simulink model "Online_Ordering_System_Functional_Architecture"  (R2025a)
settings: Solver=VariableStepAuto  StartTime=0.0  StopTime=10.0  RelTol=1e-3
model workspace (MAT data in the model file):
  Data = Simulink.Bus
  Data.Alignment = -1
  Data.PreserveElementDimensions = 0
  Data.Elements_internal(1) = Simulink.BusElement
  Data.Elements_internal(1).Min_internal = 30000
  Data.Elements_internal(1).Max_internal = 50000
  Data.Elements_internal(1).DimensionsMode = 'Fixed'
  Data.Elements_internal(1).SamplingMode = 'Sample based'
  Data.Elements_internal(1).SampleTime = -1
  Data.Elements_internal(1).Description = 'Person'
  Data.Elements_internal(1).DocUnits = '30000'
  Data.Elements_internal(1).Name = 'TargetUser'
  Data.Elements_internal(1).DataType_internal = 'single'
  Data.Elements_internal(1).Complexity = 'real'
  Data.Elements_internal(1).Dimensions = 1
  Data.Elements_internal(2) = Simulink.BusElement
  Data.Elements_internal(2).Min_internal = 10000
  Data.Elements_internal(2).Max_internal = 50000
  Data.Elements_internal(2).DimensionsMode = 'Fixed'
  Data.Elements_internal(2).SamplingMode = 'Sample based'
  Data.Elements_internal(2).SampleTime = -1
  Data.Elements_internal(2).Description = 'Person'
  Data.Elements_internal(2).DocUnits = '10000'
  Data.Elements_internal(2).Name = 'TargetPartner'
  Data.Elements_internal(2).DataType_internal = 'single'
  Data.Elements_internal(2).Complexity = 'real'
  Data.Elements_internal(2).Dimensions = 1
  Data.Elements_internal(3) = Simulink.BusElement
  Data.Elements_internal(3).Min_internal = 1
  Data.Elements_internal(3).Max_internal = 2
  Data.Elements_internal(3).DimensionsMode = 'Fixed'
  Data.Elements_internal(3).SamplingMode = 'Sample based'
  Data.Elements_internal(3).SampleTime = -1
  Data.Elements_internal(3).Description = 'Second'
  Data.Elements_internal(3).DocUnits = '2s'
  Data.Elements_internal(3).Name = 'ResponseTime'
  Data.Elements_internal(3).DataType_internal = 'single'
  Data.Elements_internal(3).Complexity = 'real'
  Data.Elements_internal(3).Dimensions = 1
  Data.Elements_internal(4) = Simulink.BusElement
  Data.Elements_internal(4).Min_internal = 1
  Data.Elements_internal(4).Max_internal = 5
  Data.Elements_internal(4).DimensionsMode = 'Fixed'
  Data.Elements_internal(4).SamplingMode = 'Sample based'
  Data.Elements_internal(4).SampleTime = -1
  Data.Elements_internal(4).Description = 'Second'
  Data.Elements_internal(4).DocUnits = '5s'
  Data.Elements_internal(4).Name = 'ProcessTime'
  Data.Elements_internal(4).DataType_internal = 'single'
  Data.Elements_internal(4).Complexity = 'real'
  Data.Elements_internal(4).Dimensions = 1
  Data.DataScope = 'Auto'
  ValueType = Simulink.ValueType
(part 1 of 2)
settings Model: Creator=OdaNobuyuki  LastModifiedBy=annic

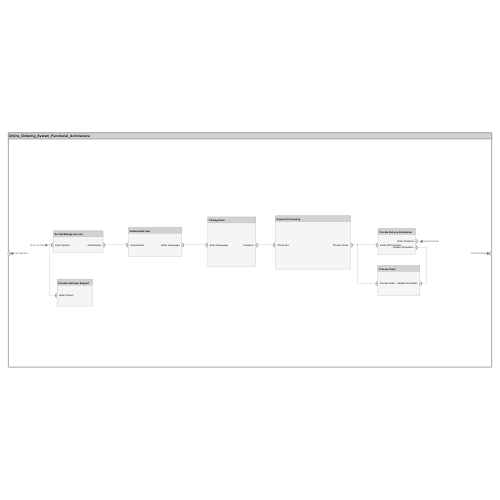
[thumbnail: Simulink's stored preview of the top-level diagram]
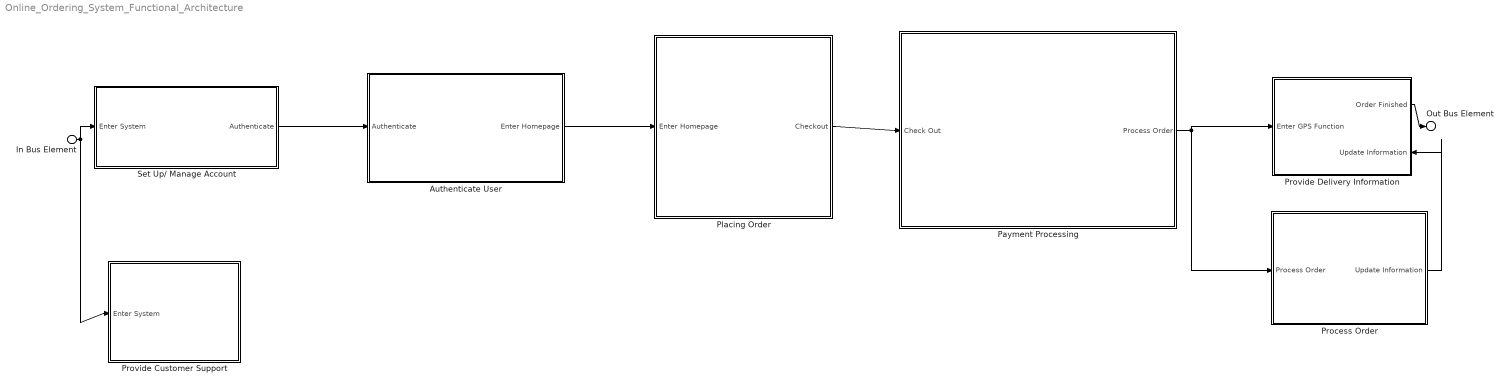
== system Online_Ordering_System_Functional_Architecture ==
  In Bus Element : Inport  PortName=Enter System
  "Authenticate User " : Subsystem
      settings: PortSchema="{\"entries\":[{\"content\":{\"headerSize\":26,\"margin\":15,\"minimumSpacing\":25,\"sides\":[{\"content\":{\"connectorIds\":[\"In1\"]},\"type\":\"ConnectorPlacement.EquallySpacedRectSide\",\"uuid\":\"427d1f3e-23ef-431e-830a-8ee80d1c0343\"},{\"content\":{\"connectorIds\":[\"Out1\"],\"side\":\"RIGHT\"},\"type\":\"ConnectorPlacement.EquallySpacedRectSide\",\"uuid\":\"a94733dc-dc80-40b7-a069-e69a5f529ec8\"},{\"content\":{\"side\":\"TOP\"},\"type\":\"ConnectorPlacement.EquallySpacedRectSide\",\"uuid\":\"aab6e856-7d0a-4bba-a547-38d5d593c589\"}]},\"type\":\"ConnectorPlacement.EquallySpacedConnector\",\"uuid\":\"17eb8191-1c5c-46d9-ae9e-c0a8464555a8\"}],\"packageUris\":[\"http://schema.mathworks.com/mf0/Connector/R2020b\"],\"version\":\"1.0\"}"
  Payment Processing : Subsystem
      settings: PortSchema="{\"entries\":[{\"content\":{\"headerSize\":26,\"margin\":15,\"minimumSpacing\":25,\"sides\":[{\"content\":{\"connectorIds\":[\"In1\"]},\"type\":\"ConnectorPlacement.EquallySpacedRectSide\",\"uuid\":\"427d1f3e-23ef-431e-830a-8ee80d1c0343\"},{\"content\":{\"connectorIds\":[\"Out1\"],\"side\":\"RIGHT\"},\"type\":\"ConnectorPlacement.EquallySpacedRectSide\",\"uuid\":\"a94733dc-dc80-40b7-a069-e69a5f529ec8\"},{\"content\":{\"side\":\"TOP\"},\"type\":\"ConnectorPlacement.EquallySpacedRectSide\",\"uuid\":\"aab6e856-7d0a-4bba-a547-38d5d593c589\"},{\"content\":{\"side\":\"BOTTOM\"},\"type\":\"ConnectorPlacement.EquallySpacedRectSide\",\"uuid\":\"c3292acf-2eb6-42cd-a4a7-82302ef25f03\"}]},\"type\":\"ConnectorPlacement.EquallySpacedConnector\",\"uuid\":\"17eb8191-1c5c-46d9-ae9e-c0a8464555a8\"}],\"packageUris\":[\"http://schema.mathworks.com/mf0/Connector/R2020b\"],\"version\":\"1.0\"}"
  Placing Order : Subsystem
      settings: PortSchema="{\"entries\":[{\"content\":{\"headerSize\":26,\"margin\":15,\"minimumSpacing\":25,\"sides\":[{\"content\":{\"connectorIds\":[\"In1\"]},\"type\":\"ConnectorPlacement.EquallySpacedRectSide\",\"uuid\":\"427d1f3e-23ef-431e-830a-8ee80d1c0343\"},{\"content\":{\"connectorIds\":[\"Out1\"],\"side\":\"RIGHT\"},\"type\":\"ConnectorPlacement.EquallySpacedRectSide\",\"uuid\":\"a94733dc-dc80-40b7-a069-e69a5f529ec8\"},{\"content\":{\"side\":\"TOP\"},\"type\":\"ConnectorPlacement.EquallySpacedRectSide\",\"uuid\":\"aab6e856-7d0a-4bba-a547-38d5d593c589\"},{\"content\":{\"side\":\"BOTTOM\"},\"type\":\"ConnectorPlacement.EquallySpacedRectSide\",\"uuid\":\"a89a1022-ae61-47b7-80bc-ebacb029706c\"}]},\"type\":\"ConnectorPlacement.EquallySpacedConnector\",\"uuid\":\"17eb8191-1c5c-46d9-ae9e-c0a8464555a8\"}],\"packageUris\":[\"http://schema.mathworks.com/mf0/Connector/R2020b\"],\"version\":\"1.0\"}"
  "Process Order " : Subsystem
      settings: PortSchema="{\"entries\":[{\"content\":{\"headerSize\":26,\"margin\":15,\"minimumSpacing\":25,\"sides\":[{\"content\":{\"connectorIds\":[\"In1\"]},\"type\":\"ConnectorPlacement.EquallySpacedRectSide\",\"uuid\":\"d2ebed04-42f4-4bd6-aa56-c214d37abe86\"},{\"content\":{\"connectorIds\":[\"Out1\"],\"side\":\"RIGHT\"},\"type\":\"ConnectorPlacement.EquallySpacedRectSide\",\"uuid\":\"0a328130-2da5-4535-b8fd-dee261bd04a3\"},{\"content\":{\"side\":\"TOP\"},\"type\":\"ConnectorPlacement.EquallySpacedRectSide\",\"uuid\":\"410ea5eb-e20b-4523-bb7e-a86253749ceb\"}]},\"type\":\"ConnectorPlacement.EquallySpacedConnector\",\"uuid\":\"5600d62f-d466-4629-981b-50f24b9b11a3\"}],\"packageUris\":[\"http://schema.mathworks.com/mf0/Connector/R2020b\"],\"version\":\"1.0\"}"
  Provide Customer Support : Subsystem
      settings: PortSchema="{\"entries\":[{\"content\":{\"headerSize\":26,\"margin\":15,\"minimumSpacing\":25,\"sides\":[{\"content\":{\"connectorIds\":[\"In1\"]},\"type\":\"ConnectorPlacement.EquallySpacedRectSide\",\"uuid\":\"427d1f3e-23ef-431e-830a-8ee80d1c0343\"},{\"content\":{\"side\":\"RIGHT\"},\"type\":\"ConnectorPlacement.EquallySpacedRectSide\",\"uuid\":\"a94733dc-dc80-40b7-a069-e69a5f529ec8\"},{\"content\":{\"side\":\"TOP\"},\"type\":\"ConnectorPlacement.EquallySpacedRectSide\",\"uuid\":\"aab6e856-7d0a-4bba-a547-38d5d593c589\"},{\"content\":{\"side\":\"BOTTOM\"},\"type\":\"ConnectorPlacement.EquallySpacedRectSide\",\"uuid\":\"351d9b7c-52a6-4554-b5b1-677764f6b427\"}]},\"type\":\"ConnectorPlacement.EquallySpacedConnector\",\"uuid\":\"17eb8191-1c5c-46d9-ae9e-c0a8464555a8\"}],\"packageUris\":[\"http://schema.mathworks.com/mf0/Connector/R2020b\"],\"version\":\"1.0\"}"
  Provide Delivery Information : Subsystem
      settings: PortSchema="{\"entries\":[{\"content\":{\"headerSize\":26,\"margin\":15,\"minimumSpacing\":25,\"sides\":[{\"content\":{\"connectorIds\":[\"In2\"]},\"type\":\"ConnectorPlacement.EquallySpacedRectSide\",\"uuid\":\"d2ebed04-42f4-4bd6-aa56-c214d37abe86\"},{\"content\":{\"connectorIds\":[\"Out1\",\"In1\"],\"side\":\"RIGHT\"},\"type\":\"ConnectorPlacement.EquallySpacedRectSide\",\"uuid\":\"0a328130-2da5-4535-b8fd-dee261bd04a3\"},{\"content\":{\"side\":\"TOP\"},\"type\":\"ConnectorPlacement.EquallySpacedRectSide\",\"uuid\":\"410ea5eb-e20b-4523-bb7e-a86253749ceb\"},{\"content\":{\"side\":\"BOTTOM\"},\"type\":\"ConnectorPlacement.EquallySpacedRectSide\",\"uuid\":\"443981ea-c855-4245-98e1-85cb0d225c25\"}]},\"type\":\"ConnectorPlacement.EquallySpacedConnector\",\"uuid\":\"5600d62f-d466-4629-981b-50f24b9b11a3\"}],\"packageUris\":[\"http://schema.mathworks.com/mf0/Connector/R2020b\"],\"version\":\"1.0\"}"
  Set Up/ Manage Account : Subsystem
      settings: PortSchema="{\"entries\":[{\"content\":{\"headerSize\":26,\"margin\":15,\"minimumSpacing\":25,\"sides\":[{\"content\":{\"connectorIds\":[\"In1\"]},\"type\":\"ConnectorPlacement.EquallySpacedRectSide\",\"uuid\":\"47f10906-199a-4fc3-b50f-b8829921055b\"},{\"content\":{\"connectorIds\":[\"Out1\"],\"side\":\"RIGHT\"},\"type\":\"ConnectorPlacement.EquallySpacedRectSide\",\"uuid\":\"92935151-f687-4cd9-918a-4edbdcb1ae87\"},{\"content\":{\"side\":\"TOP\"},\"type\":\"ConnectorPlacement.EquallySpacedRectSide\",\"uuid\":\"015ac99b-8cf7-4451-a810-2c7151c004f5\"}]},\"type\":\"ConnectorPlacement.EquallySpacedConnector\",\"uuid\":\"2d28be76-8335-46d7-935d-5d2731314622\"}],\"packageUris\":[\"http://schema.mathworks.com/mf0/Connector/R2020b\"],\"version\":\"1.0\"}"
  Out Bus Element : Outport  PortName=Order Finished
  wires:
  "Authenticate User "/1(Enter Homepage) -> Placing Order/1(Enter Homepage)
  Placing Order/1(Checkout) -> Payment Processing/1(Check Out)
  Payment Processing/1(Process Order) -> "Process Order "/1(Process Order), Provide Delivery Information/2(Enter GPS Function)
  In Bus Element/1 -> Provide Customer Support/1(Enter System), Set Up/ Manage Account/1(Enter System)
  Set Up/ Manage Account/1(Authenticate) -> "Authenticate User "/1(Authenticate)
  Provide Delivery Information/1(Order Finished) -> Out Bus Element/1
  "Process Order "/1(Update Information) -> Provide Delivery Information/1(Update Information)

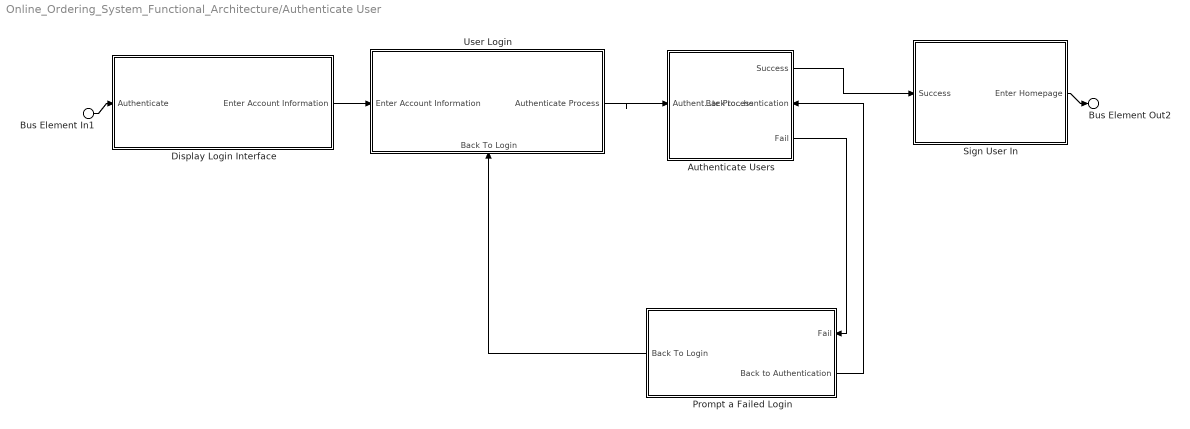
== system Online_Ordering_System_Functional_Architecture/Authenticate User  ==
  Bus Element In1 : Inport  PortName=Authenticate
  Authenticate Users : Subsystem
      settings: PortSchema="{\"entries\":[{\"content\":{\"headerSize\":26,\"margin\":15,\"minimumSpacing\":25,\"sides\":[{\"content\":{\"connectorIds\":[\"In2\"]},\"type\":\"ConnectorPlacement.EquallySpacedRectSide\",\"uuid\":\"427d1f3e-23ef-431e-830a-8ee80d1c0343\"},{\"content\":{\"connectorIds\":[\"Out1\",\"In1\",\"Out2\"],\"side\":\"RIGHT\"},\"type\":\"ConnectorPlacement.EquallySpacedRectSide\",\"uuid\":\"a94733dc-dc80-40b7-a069-e69a5f529ec8\"},{\"content\":{\"side\":\"TOP\"},\"type\":\"ConnectorPlacement.EquallySpacedRectSide\",\"uuid\":\"aab6e856-7d0a-4bba-a547-38d5d593c589\"},{\"content\":{\"side\":\"BOTTOM\"},\"type\":\"ConnectorPlacement.EquallySpacedRectSide\",\"uuid\":\"822edfb6-5de7-4787-92bc-976e01cc291a\"}]},\"type\":\"ConnectorPlacement.EquallySpacedConnector\",\"uuid\":\"17eb8191-1c5c-46d9-ae9e-c0a8464555a8\"}],\"packageUris\":[\"http://schema.mathworks.com/mf0/Connector/R2020b\"],\"version\":\"1.0\"}"
  Display Login Interface : Subsystem
      settings: PortSchema="{\"entries\":[{\"content\":{\"headerSize\":26,\"margin\":15,\"minimumSpacing\":25,\"sides\":[{\"content\":{\"connectorIds\":[\"In1\"]},\"type\":\"ConnectorPlacement.EquallySpacedRectSide\",\"uuid\":\"cbb74984-7595-4789-b046-96ead26edeb9\"},{\"content\":{\"connectorIds\":[\"Out1\"],\"side\":\"RIGHT\"},\"type\":\"ConnectorPlacement.EquallySpacedRectSide\",\"uuid\":\"b6bb8368-8099-4b12-9d55-2c29ae804ffc\"},{\"content\":{\"side\":\"TOP\"},\"type\":\"ConnectorPlacement.EquallySpacedRectSide\",\"uuid\":\"14a6774e-c600-4f70-83e3-a7d0c3cf7479\"},{\"content\":{\"side\":\"BOTTOM\"},\"type\":\"ConnectorPlacement.EquallySpacedRectSide\",\"uuid\":\"deb2294e-400e-4f84-ba24-f2715792f4b9\"}]},\"type\":\"ConnectorPlacement.EquallySpacedConnector\",\"uuid\":\"469ef3cc-c012-4ecc-a677-bf3638dfce1b\"}],\"packageUris\":[\"http://schema.mathworks.com/mf0/Connector/R2020b\"],\"version\":\"1.0\"}"
  Prompt a Failed Login : Subsystem
      settings: PortSchema="{\"entries\":[{\"content\":{\"headerSize\":26,\"margin\":15,\"minimumSpacing\":25,\"sides\":[{\"content\":{\"connectorIds\":[\"Out1\"]},\"type\":\"ConnectorPlacement.EquallySpacedRectSide\",\"uuid\":\"427d1f3e-23ef-431e-830a-8ee80d1c0343\"},{\"content\":{\"connectorIds\":[\"In1\",\"Out2\"],\"side\":\"RIGHT\"},\"type\":\"ConnectorPlacement.EquallySpacedRectSide\",\"uuid\":\"a94733dc-dc80-40b7-a069-e69a5f529ec8\"},{\"content\":{\"side\":\"TOP\"},\"type\":\"ConnectorPlacement.EquallySpacedRectSide\",\"uuid\":\"aab6e856-7d0a-4bba-a547-38d5d593c589\"}]},\"type\":\"ConnectorPlacement.EquallySpacedConnector\",\"uuid\":\"17eb8191-1c5c-46d9-ae9e-c0a8464555a8\"}],\"packageUris\":[\"http://schema.mathworks.com/mf0/Connector/R2020b\"],\"version\":\"1.0\"}"
  Sign User In : Subsystem
      settings: PortSchema="{\"entries\":[{\"content\":{\"headerSize\":26,\"margin\":15,\"minimumSpacing\":25,\"sides\":[{\"content\":{\"connectorIds\":[\"In1\"]},\"type\":\"ConnectorPlacement.EquallySpacedRectSide\",\"uuid\":\"427d1f3e-23ef-431e-830a-8ee80d1c0343\"},{\"content\":{\"connectorIds\":[\"Out1\"],\"side\":\"RIGHT\"},\"type\":\"ConnectorPlacement.EquallySpacedRectSide\",\"uuid\":\"a94733dc-dc80-40b7-a069-e69a5f529ec8\"},{\"content\":{\"side\":\"TOP\"},\"type\":\"ConnectorPlacement.EquallySpacedRectSide\",\"uuid\":\"aab6e856-7d0a-4bba-a547-38d5d593c589\"},{\"content\":{\"side\":\"BOTTOM\"},\"type\":\"ConnectorPlacement.EquallySpacedRectSide\",\"uuid\":\"4782b0d4-0180-487e-b6f5-72f073cbe76a\"}]},\"type\":\"ConnectorPlacement.EquallySpacedConnector\",\"uuid\":\"17eb8191-1c5c-46d9-ae9e-c0a8464555a8\"}],\"packageUris\":[\"http://schema.mathworks.com/mf0/Connector/R2020b\"],\"version\":\"1.0\"}"
  "User Login " : Subsystem
      settings: PortSchema="{\"entries\":[{\"content\":{\"headerSize\":26,\"margin\":15,\"minimumSpacing\":25,\"sides\":[{\"content\":{\"connectorIds\":[\"In2\"]},\"type\":\"ConnectorPlacement.EquallySpacedRectSide\",\"uuid\":\"d2ebed04-42f4-4bd6-aa56-c214d37abe86\"},{\"content\":{\"connectorIds\":[\"Out1\"],\"side\":\"RIGHT\"},\"type\":\"ConnectorPlacement.EquallySpacedRectSide\",\"uuid\":\"0a328130-2da5-4535-b8fd-dee261bd04a3\"},{\"content\":{\"side\":\"TOP\"},\"type\":\"ConnectorPlacement.EquallySpacedRectSide\",\"uuid\":\"410ea5eb-e20b-4523-bb7e-a86253749ceb\"},{\"content\":{\"connectorIds\":[\"In1\"],\"side\":\"BOTTOM\"},\"type\":\"ConnectorPlacement.EquallySpacedRectSide\",\"uuid\":\"388ab0ab-6a87-40e3-b544-46c520a133d8\"}]},\"type\":\"ConnectorPlacement.EquallySpacedConnector\",\"uuid\":\"5600d62f-d466-4629-981b-50f24b9b11a3\"}],\"packageUris\":[\"http://schema.mathworks.com/mf0/Connector/R2020b\"],\"version\":\"1.0\"}"
  Bus Element Out2 : Outport  PortName=Enter Homepage
  wires:
  Authenticate Users/1(Success) -> Sign User In/1(Success)
  Display Login Interface/1(Enter Account Information) -> "User Login "/2(Enter Account Information)
  Prompt a Failed Login/2(Back to Authentication) -> Authenticate Users/1(Back to Authentication)
  "User Login "/1(Authenticate Process) -> Authenticate Users/2(Authenticate Process)
  Prompt a Failed Login/1(Back To Login) -> "User Login "/1(Back To Login)
  Sign User In/1(Enter Homepage) -> Bus Element Out2/1
  Bus Element In1/1 -> Display Login Interface/1(Authenticate)
  Authenticate Users/2(Fail) -> Prompt a Failed Login/1(Fail)

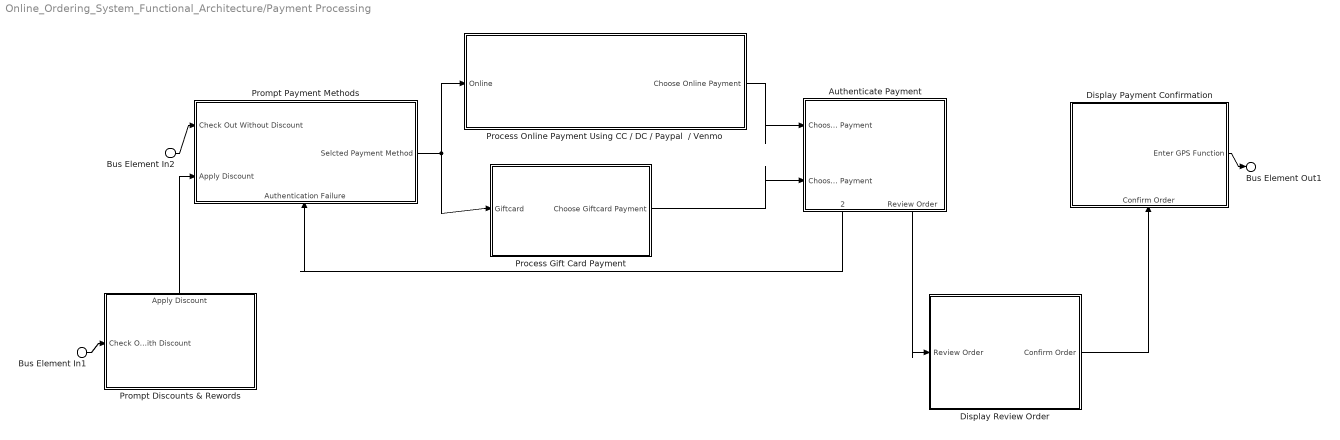
== system Online_Ordering_System_Functional_Architecture/Payment Processing ==
  Bus Element In1 : Inport  PortName=Check Out
  Bus Element In2 : Inport  PortName=Check Out
  Authenticate Payment : Subsystem
      settings: PortSchema="{\"entries\":[{\"content\":{\"headerSize\":26,\"margin\":15,\"minimumSpacing\":25,\"sides\":[{\"content\":{\"connectorIds\":[\"In1\",\"In2\"]},\"type\":\"ConnectorPlacement.EquallySpacedRectSide\",\"uuid\":\"427d1f3e-23ef-431e-830a-8ee80d1c0343\"},{\"content\":{\"side\":\"RIGHT\"},\"type\":\"ConnectorPlacement.EquallySpacedRectSide\",\"uuid\":\"a94733dc-dc80-40b7-a069-e69a5f529ec8\"},{\"content\":{\"side\":\"TOP\"},\"type\":\"ConnectorPlacement.EquallySpacedRectSide\",\"uuid\":\"aab6e856-7d0a-4bba-a547-38d5d593c589\"},{\"content\":{\"connectorIds\":[\"Out2\",\"Out1\"],\"side\":\"BOTTOM\"},\"type\":\"ConnectorPlacement.EquallySpacedRectSide\",\"uuid\":\"2134340b-1a1d-4804-aa4c-47d156557184\"}]},\"type\":\"ConnectorPlacement.EquallySpacedConnector\",\"uuid\":\"17eb8191-1c5c-46d9-ae9e-c0a8464555a8\"}],\"packageUris\":[\"http://schema.mathworks.com/mf0/Connector/R2020b\"],\"version\":\"1.0\"}"
  Display Payment Confirmation : Subsystem
      settings: PortSchema="{\"entries\":[{\"content\":{\"headerSize\":26,\"margin\":15,\"minimumSpacing\":25,\"sides\":[{\"content\":{},\"type\":\"ConnectorPlacement.EquallySpacedRectSide\",\"uuid\":\"cbb74984-7595-4789-b046-96ead26edeb9\"},{\"content\":{\"connectorIds\":[\"Out1\"],\"side\":\"RIGHT\"},\"type\":\"ConnectorPlacement.EquallySpacedRectSide\",\"uuid\":\"b6bb8368-8099-4b12-9d55-2c29ae804ffc\"},{\"content\":{\"side\":\"TOP\"},\"type\":\"ConnectorPlacement.EquallySpacedRectSide\",\"uuid\":\"14a6774e-c600-4f70-83e3-a7d0c3cf7479\"},{\"content\":{\"connectorIds\":[\"In1\"],\"side\":\"BOTTOM\"},\"type\":\"ConnectorPlacement.EquallySpacedRectSide\",\"uuid\":\"a82d93e2-79e4-4503-92a2-65c1f83a9361\"}]},\"type\":\"ConnectorPlacement.EquallySpacedConnector\",\"uuid\":\"469ef3cc-c012-4ecc-a677-bf3638dfce1b\"}],\"packageUris\":[\"http://schema.mathworks.com/mf0/Connector/R2020b\"],\"version\":\"1.0\"}"
  Display Review Order : Subsystem
      settings: PortSchema="{\"entries\":[{\"content\":{\"headerSize\":26,\"margin\":15,\"minimumSpacing\":25,\"sides\":[{\"content\":{\"connectorIds\":[\"In1\"]},\"type\":\"ConnectorPlacement.EquallySpacedRectSide\",\"uuid\":\"47f10906-199a-4fc3-b50f-b8829921055b\"},{\"content\":{\"connectorIds\":[\"Out1\"],\"side\":\"RIGHT\"},\"type\":\"ConnectorPlacement.EquallySpacedRectSide\",\"uuid\":\"92935151-f687-4cd9-918a-4edbdcb1ae87\"},{\"content\":{\"side\":\"TOP\"},\"type\":\"ConnectorPlacement.EquallySpacedRectSide\",\"uuid\":\"015ac99b-8cf7-4451-a810-2c7151c004f5\"}]},\"type\":\"ConnectorPlacement.EquallySpacedConnector\",\"uuid\":\"2d28be76-8335-46d7-935d-5d2731314622\"}],\"packageUris\":[\"http://schema.mathworks.com/mf0/Connector/R2020b\"],\"version\":\"1.0\"}"
  Process Gift Card Payment : Subsystem
      settings: PortSchema="{\"entries\":[{\"content\":{\"headerSize\":26,\"margin\":15,\"minimumSpacing\":25,\"sides\":[{\"content\":{\"connectorIds\":[\"In1\"]},\"type\":\"ConnectorPlacement.EquallySpacedRectSide\",\"uuid\":\"427d1f3e-23ef-431e-830a-8ee80d1c0343\"},{\"content\":{\"connectorIds\":[\"Out1\"],\"side\":\"RIGHT\"},\"type\":\"ConnectorPlacement.EquallySpacedRectSide\",\"uuid\":\"a94733dc-dc80-40b7-a069-e69a5f529ec8\"},{\"content\":{\"side\":\"TOP\"},\"type\":\"ConnectorPlacement.EquallySpacedRectSide\",\"uuid\":\"aab6e856-7d0a-4bba-a547-38d5d593c589\"}]},\"type\":\"ConnectorPlacement.EquallySpacedConnector\",\"uuid\":\"17eb8191-1c5c-46d9-ae9e-c0a8464555a8\"}],\"packageUris\":[\"http://schema.mathworks.com/mf0/Connector/R2020b\"],\"version\":\"1.0\"}"
  Process Online Payment Using CC / DC / Paypal  / Venmo : Subsystem
      settings: PortSchema="{\"entries\":[{\"content\":{\"headerSize\":26,\"margin\":15,\"minimumSpacing\":25,\"sides\":[{\"content\":{\"connectorIds\":[\"In1\"]},\"type\":\"ConnectorPlacement.EquallySpacedRectSide\",\"uuid\":\"427d1f3e-23ef-431e-830a-8ee80d1c0343\"},{\"content\":{\"connectorIds\":[\"Out1\"],\"side\":\"RIGHT\"},\"type\":\"ConnectorPlacement.EquallySpacedRectSide\",\"uuid\":\"a94733dc-dc80-40b7-a069-e69a5f529ec8\"},{\"content\":{\"side\":\"TOP\"},\"type\":\"ConnectorPlacement.EquallySpacedRectSide\",\"uuid\":\"aab6e856-7d0a-4bba-a547-38d5d593c589\"}]},\"type\":\"ConnectorPlacement.EquallySpacedConnector\",\"uuid\":\"17eb8191-1c5c-46d9-ae9e-c0a8464555a8\"}],\"packageUris\":[\"http://schema.mathworks.com/mf0/Connector/R2020b\"],\"version\":\"1.0\"}"
  Prompt Discounts & Rewords : Subsystem
      settings: PortSchema="{\"entries\":[{\"content\":{\"headerSize\":26,\"margin\":15,\"minimumSpacing\":25,\"sides\":[{\"content\":{\"connectorIds\":[\"In1\"]},\"type\":\"ConnectorPlacement.EquallySpacedRectSide\",\"uuid\":\"427d1f3e-23ef-431e-830a-8ee80d1c0343\"},{\"content\":{\"side\":\"RIGHT\"},\"type\":\"ConnectorPlacement.EquallySpacedRectSide\",\"uuid\":\"a94733dc-dc80-40b7-a069-e69a5f529ec8\"},{\"content\":{\"connectorIds\":[\"Out1\"],\"side\":\"TOP\"},\"type\":\"ConnectorPlacement.EquallySpacedRectSide\",\"uuid\":\"aab6e856-7d0a-4bba-a547-38d5d593c589\"}]},\"type\":\"ConnectorPlacement.EquallySpacedConnector\",\"uuid\":\"17eb8191-1c5c-46d9-ae9e-c0a8464555a8\"}],\"packageUris\":[\"http://schema.mathworks.com/mf0/Connector/R2020b\"],\"version\":\"1.0\"}"
  Prompt Payment Methods : Subsystem
      settings: PortSchema="{\"entries\":[{\"content\":{\"headerSize\":26,\"margin\":15,\"minimumSpacing\":25,\"sides\":[{\"content\":{\"connectorIds\":[\"In1\",\"In2\"]},\"type\":\"ConnectorPlacement.EquallySpacedRectSide\",\"uuid\":\"427d1f3e-23ef-431e-830a-8ee80d1c0343\"},{\"content\":{\"connectorIds\":[\"Out1\"],\"side\":\"RIGHT\"},\"type\":\"ConnectorPlacement.EquallySpacedRectSide\",\"uuid\":\"a94733dc-dc80-40b7-a069-e69a5f529ec8\"},{\"content\":{\"side\":\"TOP\"},\"type\":\"ConnectorPlacement.EquallySpacedRectSide\",\"uuid\":\"aab6e856-7d0a-4bba-a547-38d5d593c589\"},{\"content\":{\"connectorIds\":[\"In3\"],\"side\":\"BOTTOM\"},\"type\":\"ConnectorPlacement.EquallySpacedRectSide\",\"uuid\":\"301fbdec-26db-4103-a088-b13178cf7d4f\"}]},\"type\":\"ConnectorPlacement.EquallySpacedConnector\",\"uuid\":\"17eb8191-1c5c-46d9-ae9e-c0a8464555a8\"}],\"packageUris\":[\"http://schema.mathworks.com/mf0/Connector/R2020b\"],\"version\":\"1.0\"}"
  Bus Element Out1 : Outport  PortName=Process Order
  wires:
  Prompt Payment Methods/1(Selcted Payment Method) -> Process Online Payment Using CC / DC / Paypal  / Venmo/1(Online), Process Gift Card Payment/1(Giftcard)
  Process Online Payment Using CC / DC / Paypal  / Venmo/1(Choose Online Payment) -> Authenticate Payment/1(Choose Online Payment)
  Process Gift Card Payment/1(Choose Giftcard Payment) -> Authenticate Payment/2(Choose Giftcard Payment)
  Authenticate Payment/2(Authentication Failure) -> Prompt Payment Methods/3(Authentication Failure)
  Bus Element In1/1 -> Prompt Discounts & Rewords/1(Check Out With Discount)
  Prompt Discounts & Rewords/1(Apply Discount) -> Prompt Payment Methods/2(Apply Discount)
  Bus Element In2/1 -> Prompt Payment Methods/1(Check Out Without Discount)
  Authenticate Payment/1(Review Order) -> Display Review Order/1(Review Order)
  Display Review Order/1(Confirm Order) -> Display Payment Confirmation/1(Confirm Order)
  Display Payment Confirmation/1(Enter GPS Function) -> Bus Element Out1/1

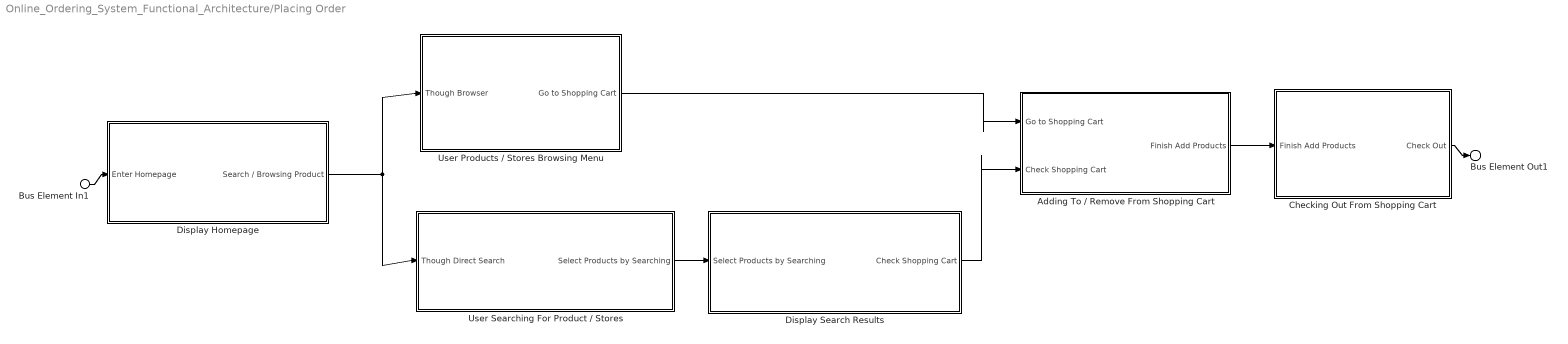
== system Online_Ordering_System_Functional_Architecture/Placing Order ==
  Bus Element In1 : Inport  PortName=Enter Homepage
  "Adding To / Remove From Shopping Cart " : Subsystem
      settings: PortSchema="{\"entries\":[{\"content\":{\"headerSize\":26,\"margin\":15,\"minimumSpacing\":25,\"sides\":[{\"content\":{\"connectorIds\":[\"In1\",\"In2\"]},\"type\":\"ConnectorPlacement.EquallySpacedRectSide\",\"uuid\":\"427d1f3e-23ef-431e-830a-8ee80d1c0343\"},{\"content\":{\"connectorIds\":[\"Out1\"],\"side\":\"RIGHT\"},\"type\":\"ConnectorPlacement.EquallySpacedRectSide\",\"uuid\":\"a94733dc-dc80-40b7-a069-e69a5f529ec8\"},{\"content\":{\"side\":\"TOP\"},\"type\":\"ConnectorPlacement.EquallySpacedRectSide\",\"uuid\":\"aab6e856-7d0a-4bba-a547-38d5d593c589\"},{\"content\":{\"side\":\"BOTTOM\"},\"type\":\"ConnectorPlacement.EquallySpacedRectSide\",\"uuid\":\"b903f41b-b4dc-49c0-8a4d-a823a8bb045a\"}]},\"type\":\"ConnectorPlacement.EquallySpacedConnector\",\"uuid\":\"17eb8191-1c5c-46d9-ae9e-c0a8464555a8\"}],\"packageUris\":[\"http://schema.mathworks.com/mf0/Connector/R2020b\"],\"version\":\"1.0\"}"
  Checking Out From Shopping Cart : Subsystem
      settings: PortSchema="{\"entries\":[{\"content\":{\"headerSize\":26,\"margin\":15,\"minimumSpacing\":25,\"sides\":[{\"content\":{\"connectorIds\":[\"In1\"]},\"type\":\"ConnectorPlacement.EquallySpacedRectSide\",\"uuid\":\"d2ebed04-42f4-4bd6-aa56-c214d37abe86\"},{\"content\":{\"connectorIds\":[\"Out1\"],\"side\":\"RIGHT\"},\"type\":\"ConnectorPlacement.EquallySpacedRectSide\",\"uuid\":\"0a328130-2da5-4535-b8fd-dee261bd04a3\"},{\"content\":{\"side\":\"TOP\"},\"type\":\"ConnectorPlacement.EquallySpacedRectSide\",\"uuid\":\"410ea5eb-e20b-4523-bb7e-a86253749ceb\"}]},\"type\":\"ConnectorPlacement.EquallySpacedConnector\",\"uuid\":\"5600d62f-d466-4629-981b-50f24b9b11a3\"}],\"packageUris\":[\"http://schema.mathworks.com/mf0/Connector/R2020b\"],\"version\":\"1.0\"}"
  Display Homepage : Subsystem
      settings: PortSchema="{\"entries\":[{\"content\":{\"headerSize\":26,\"margin\":15,\"minimumSpacing\":25,\"sides\":[{\"content\":{\"connectorIds\":[\"In1\"]},\"type\":\"ConnectorPlacement.EquallySpacedRectSide\",\"uuid\":\"cbb74984-7595-4789-b046-96ead26edeb9\"},{\"content\":{\"connectorIds\":[\"Out1\"],\"side\":\"RIGHT\"},\"type\":\"ConnectorPlacement.EquallySpacedRectSide\",\"uuid\":\"b6bb8368-8099-4b12-9d55-2c29ae804ffc\"},{\"content\":{\"side\":\"TOP\"},\"type\":\"ConnectorPlacement.EquallySpacedRectSide\",\"uuid\":\"14a6774e-c600-4f70-83e3-a7d0c3cf7479\"},{\"content\":{\"side\":\"BOTTOM\"},\"type\":\"ConnectorPlacement.EquallySpacedRectSide\",\"uuid\":\"d057ab6e-a0b6-4baa-a98f-672ff88698d4\"}]},\"type\":\"ConnectorPlacement.EquallySpacedConnector\",\"uuid\":\"469ef3cc-c012-4ecc-a677-bf3638dfce1b\"}],\"packageUris\":[\"http://schema.mathworks.com/mf0/Connector/R2020b\"],\"version\":\"1.0\"}"
  Display Search Results : Subsystem
      settings: PortSchema="{\"entries\":[{\"content\":{\"headerSize\":26,\"margin\":15,\"minimumSpacing\":25,\"sides\":[{\"content\":{\"connectorIds\":[\"In1\"]},\"type\":\"ConnectorPlacement.EquallySpacedRectSide\",\"uuid\":\"cbb74984-7595-4789-b046-96ead26edeb9\"},{\"content\":{\"connectorIds\":[\"Out1\"],\"side\":\"RIGHT\"},\"type\":\"ConnectorPlacement.EquallySpacedRectSide\",\"uuid\":\"b6bb8368-8099-4b12-9d55-2c29ae804ffc\"},{\"content\":{\"side\":\"TOP\"},\"type\":\"ConnectorPlacement.EquallySpacedRectSide\",\"uuid\":\"14a6774e-c600-4f70-83e3-a7d0c3cf7479\"},{\"content\":{\"side\":\"BOTTOM\"},\"type\":\"ConnectorPlacement.EquallySpacedRectSide\",\"uuid\":\"96a52d4b-311b-45a3-8c8a-5b70822256d6\"}]},\"type\":\"ConnectorPlacement.EquallySpacedConnector\",\"uuid\":\"469ef3cc-c012-4ecc-a677-bf3638dfce1b\"}],\"packageUris\":[\"http://schema.mathworks.com/mf0/Connector/R2020b\"],\"version\":\"1.0\"}"
  User Products / Stores Browsing Menu : Subsystem
      settings: PortSchema="{\"entries\":[{\"content\":{\"headerSize\":26,\"margin\":15,\"minimumSpacing\":25,\"sides\":[{\"content\":{\"connectorIds\":[\"In1\"]},\"type\":\"ConnectorPlacement.EquallySpacedRectSide\",\"uuid\":\"427d1f3e-23ef-431e-830a-8ee80d1c0343\"},{\"content\":{\"connectorIds\":[\"Out1\"],\"side\":\"RIGHT\"},\"type\":\"ConnectorPlacement.EquallySpacedRectSide\",\"uuid\":\"a94733dc-dc80-40b7-a069-e69a5f529ec8\"},{\"content\":{\"side\":\"TOP\"},\"type\":\"ConnectorPlacement.EquallySpacedRectSide\",\"uuid\":\"aab6e856-7d0a-4bba-a547-38d5d593c589\"},{\"content\":{\"side\":\"BOTTOM\"},\"type\":\"ConnectorPlacement.EquallySpacedRectSide\",\"uuid\":\"06e25ceb-3515-4a34-9a5e-b52bdfde88f0\"}]},\"type\":\"ConnectorPlacement.EquallySpacedConnector\",\"uuid\":\"17eb8191-1c5c-46d9-ae9e-c0a8464555a8\"}],\"packageUris\":[\"http://schema.mathworks.com/mf0/Connector/R2020b\"],\"version\":\"1.0\"}"
  User Searching For Product / Stores : Subsystem
      settings: PortSchema="{\"entries\":[{\"content\":{\"headerSize\":26,\"margin\":15,\"minimumSpacing\":25,\"sides\":[{\"content\":{\"connectorIds\":[\"In1\"]},\"type\":\"ConnectorPlacement.EquallySpacedRectSide\",\"uuid\":\"427d1f3e-23ef-431e-830a-8ee80d1c0343\"},{\"content\":{\"connectorIds\":[\"Out1\"],\"side\":\"RIGHT\"},\"type\":\"ConnectorPlacement.EquallySpacedRectSide\",\"uuid\":\"a94733dc-dc80-40b7-a069-e69a5f529ec8\"},{\"content\":{\"side\":\"TOP\"},\"type\":\"ConnectorPlacement.EquallySpacedRectSide\",\"uuid\":\"aab6e856-7d0a-4bba-a547-38d5d593c589\"},{\"content\":{\"side\":\"BOTTOM\"},\"type\":\"ConnectorPlacement.EquallySpacedRectSide\",\"uuid\":\"442269c5-54c2-4a2e-b298-a7048d1c7a55\"}]},\"type\":\"ConnectorPlacement.EquallySpacedConnector\",\"uuid\":\"17eb8191-1c5c-46d9-ae9e-c0a8464555a8\"}],\"packageUris\":[\"http://schema.mathworks.com/mf0/Connector/R2020b\"],\"version\":\"1.0\"}"
  Bus Element Out1 : Outport  PortName=Checkout
  wires:
  Display Homepage/1(Search / Browsing Product) -> User Products / Stores Browsing Menu/1(Though Browser), User Searching For Product / Stores/1(Though Direct Search)
  User Searching For Product / Stores/1(Select Products by Searching) -> Display Search Results/1(Select Products by Searching)
  Display Search Results/1(Check Shopping Cart) -> "Adding To / Remove From Shopping Cart "/2(Check Shopping Cart)
  Bus Element In1/1 -> Display Homepage/1(Enter Homepage)
  User Products / Stores Browsing Menu/1(Go to Shopping Cart) -> "Adding To / Remove From Shopping Cart "/1(Go to Shopping Cart)
  "Adding To / Remove From Shopping Cart "/1(Finish Add Products) -> Checking Out From Shopping Cart/1(Finish Add Products)
  Checking Out From Shopping Cart/1(Check Out) -> Bus Element Out1/1

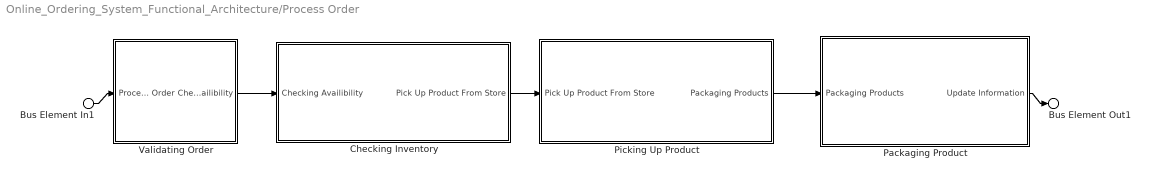
== system Online_Ordering_System_Functional_Architecture/Process Order  ==
  Bus Element In1 : Inport  PortName=Process Order
  Checking Inventory : Subsystem
      settings: PortSchema="{\"entries\":[{\"content\":{\"headerSize\":26,\"margin\":15,\"minimumSpacing\":25,\"sides\":[{\"content\":{\"connectorIds\":[\"In1\"]},\"type\":\"ConnectorPlacement.EquallySpacedRectSide\",\"uuid\":\"d2ebed04-42f4-4bd6-aa56-c214d37abe86\"},{\"content\":{\"connectorIds\":[\"Out1\"],\"side\":\"RIGHT\"},\"type\":\"ConnectorPlacement.EquallySpacedRectSide\",\"uuid\":\"0a328130-2da5-4535-b8fd-dee261bd04a3\"},{\"content\":{\"side\":\"TOP\"},\"type\":\"ConnectorPlacement.EquallySpacedRectSide\",\"uuid\":\"410ea5eb-e20b-4523-bb7e-a86253749ceb\"}]},\"type\":\"ConnectorPlacement.EquallySpacedConnector\",\"uuid\":\"5600d62f-d466-4629-981b-50f24b9b11a3\"}],\"packageUris\":[\"http://schema.mathworks.com/mf0/Connector/R2020b\"],\"version\":\"1.0\"}"
  Packaging Product : Subsystem
      settings: PortSchema="{\"entries\":[{\"content\":{\"headerSize\":26,\"margin\":15,\"minimumSpacing\":25,\"sides\":[{\"content\":{\"connectorIds\":[\"In1\"]},\"type\":\"ConnectorPlacement.EquallySpacedRectSide\",\"uuid\":\"d2ebed04-42f4-4bd6-aa56-c214d37abe86\"},{\"content\":{\"connectorIds\":[\"Out1\"],\"side\":\"RIGHT\"},\"type\":\"ConnectorPlacement.EquallySpacedRectSide\",\"uuid\":\"0a328130-2da5-4535-b8fd-dee261bd04a3\"},{\"content\":{\"side\":\"TOP\"},\"type\":\"ConnectorPlacement.EquallySpacedRectSide\",\"uuid\":\"410ea5eb-e20b-4523-bb7e-a86253749ceb\"}]},\"type\":\"ConnectorPlacement.EquallySpacedConnector\",\"uuid\":\"5600d62f-d466-4629-981b-50f24b9b11a3\"}],\"packageUris\":[\"http://schema.mathworks.com/mf0/Connector/R2020b\"],\"version\":\"1.0\"}"
  Picking Up Product : Subsystem
      settings: PortSchema="{\"entries\":[{\"content\":{\"headerSize\":26,\"margin\":15,\"minimumSpacing\":25,\"sides\":[{\"content\":{\"connectorIds\":[\"In1\"]},\"type\":\"ConnectorPlacement.EquallySpacedRectSide\",\"uuid\":\"d2ebed04-42f4-4bd6-aa56-c214d37abe86\"},{\"content\":{\"connectorIds\":[\"Out1\"],\"side\":\"RIGHT\"},\"type\":\"ConnectorPlacement.EquallySpacedRectSide\",\"uuid\":\"0a328130-2da5-4535-b8fd-dee261bd04a3\"},{\"content\":{\"side\":\"TOP\"},\"type\":\"ConnectorPlacement.EquallySpacedRectSide\",\"uuid\":\"410ea5eb-e20b-4523-bb7e-a86253749ceb\"}]},\"type\":\"ConnectorPlacement.EquallySpacedConnector\",\"uuid\":\"5600d62f-d466-4629-981b-50f24b9b11a3\"}],\"packageUris\":[\"http://schema.mathworks.com/mf0/Connector/R2020b\"],\"version\":\"1.0\"}"
  Validating Order : Subsystem
      settings: PortSchema="{\"entries\":[{\"content\":{\"headerSize\":26,\"margin\":15,\"minimumSpacing\":25,\"sides\":[{\"content\":{\"connectorIds\":[\"In1\"]},\"type\":\"ConnectorPlacement.EquallySpacedRectSide\",\"uuid\":\"d2ebed04-42f4-4bd6-aa56-c214d37abe86\"},{\"content\":{\"connectorIds\":[\"Out1\"],\"side\":\"RIGHT\"},\"type\":\"ConnectorPlacement.EquallySpacedRectSide\",\"uuid\":\"0a328130-2da5-4535-b8fd-dee261bd04a3\"},{\"content\":{\"side\":\"TOP\"},\"type\":\"ConnectorPlacement.EquallySpacedRectSide\",\"uuid\":\"410ea5eb-e20b-4523-bb7e-a86253749ceb\"}]},\"type\":\"ConnectorPlacement.EquallySpacedConnector\",\"uuid\":\"5600d62f-d466-4629-981b-50f24b9b11a3\"}],\"packageUris\":[\"http://schema.mathworks.com/mf0/Connector/R2020b\"],\"version\":\"1.0\"}"
  Bus Element Out1 : Outport  PortName=Update Information
  wires:
  Validating Order/1("Checking Availibility ") -> Checking Inventory/1("Checking Availibility ")
  Checking Inventory/1(Pick Up Product From Store) -> Picking Up Product/1(Pick Up Product From Store)
  Picking Up Product/1(Packaging Products) -> Packaging Product/1(Packaging Products)
  Packaging Product/1(Update Information) -> Bus Element Out1/1
  Bus Element In1/1 -> Validating Order/1(Process Order)

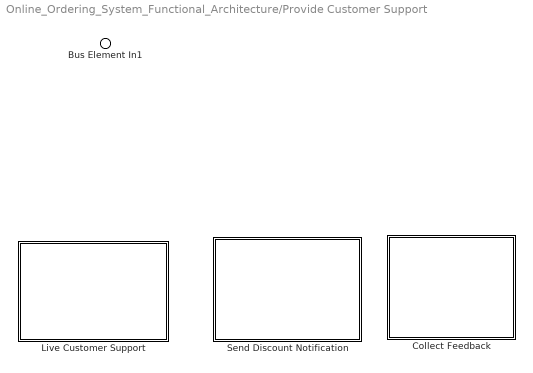
== system Online_Ordering_System_Functional_Architecture/Provide Customer Support ==
  Bus Element In1 : Inport  PortName=Enter System
  Collect Feedback : Subsystem
      settings: PortSchema="{\"entries\":[{\"content\":{\"headerSize\":26,\"margin\":15,\"minimumSpacing\":25,\"sides\":[{\"content\":{},\"type\":\"ConnectorPlacement.EquallySpacedRectSide\",\"uuid\":\"47f10906-199a-4fc3-b50f-b8829921055b\"},{\"content\":{\"side\":\"RIGHT\"},\"type\":\"ConnectorPlacement.EquallySpacedRectSide\",\"uuid\":\"92935151-f687-4cd9-918a-4edbdcb1ae87\"},{\"content\":{\"side\":\"TOP\"},\"type\":\"ConnectorPlacement.EquallySpacedRectSide\",\"uuid\":\"015ac99b-8cf7-4451-a810-2c7151c004f5\"},{\"content\":{\"side\":\"BOTTOM\"},\"type\":\"ConnectorPlacement.EquallySpacedRectSide\",\"uuid\":\"eec9be38-4ba6-426b-a1f1-2c37e91dc163\"}]},\"type\":\"ConnectorPlacement.EquallySpacedConnector\",\"uuid\":\"2d28be76-8335-46d7-935d-5d2731314622\"}],\"packageUris\":[\"http://schema.mathworks.com/mf0/Connector/R2020b\"],\"version\":\"1.0\"}"
  Live Customer Support : Subsystem
      settings: PortSchema="{\"entries\":[{\"content\":{\"headerSize\":26,\"margin\":15,\"minimumSpacing\":25,\"sides\":[{\"content\":{},\"type\":\"ConnectorPlacement.EquallySpacedRectSide\",\"uuid\":\"47f10906-199a-4fc3-b50f-b8829921055b\"},{\"content\":{\"side\":\"RIGHT\"},\"type\":\"ConnectorPlacement.EquallySpacedRectSide\",\"uuid\":\"92935151-f687-4cd9-918a-4edbdcb1ae87\"},{\"content\":{\"side\":\"TOP\"},\"type\":\"ConnectorPlacement.EquallySpacedRectSide\",\"uuid\":\"015ac99b-8cf7-4451-a810-2c7151c004f5\"},{\"content\":{\"side\":\"BOTTOM\"},\"type\":\"ConnectorPlacement.EquallySpacedRectSide\",\"uuid\":\"c8e12821-783c-47e1-bb50-05fb22703402\"}]},\"type\":\"ConnectorPlacement.EquallySpacedConnector\",\"uuid\":\"2d28be76-8335-46d7-935d-5d2731314622\"}],\"packageUris\":[\"http://schema.mathworks.com/mf0/Connector/R2020b\"],\"version\":\"1.0\"}"
  Send Discount Notification : Subsystem
      settings: PortSchema="{\"entries\":[{\"content\":{\"headerSize\":26,\"margin\":15,\"minimumSpacing\":25,\"sides\":[{\"content\":{},\"type\":\"ConnectorPlacement.EquallySpacedRectSide\",\"uuid\":\"47f10906-199a-4fc3-b50f-b8829921055b\"},{\"content\":{\"side\":\"RIGHT\"},\"type\":\"ConnectorPlacement.EquallySpacedRectSide\",\"uuid\":\"92935151-f687-4cd9-918a-4edbdcb1ae87\"},{\"content\":{\"side\":\"TOP\"},\"type\":\"ConnectorPlacement.EquallySpacedRectSide\",\"uuid\":\"015ac99b-8cf7-4451-a810-2c7151c004f5\"},{\"content\":{\"side\":\"BOTTOM\"},\"type\":\"ConnectorPlacement.EquallySpacedRectSide\",\"uuid\":\"ba1e2227-187e-420e-b74b-a66b6d876499\"}]},\"type\":\"ConnectorPlacement.EquallySpacedConnector\",\"uuid\":\"2d28be76-8335-46d7-935d-5d2731314622\"}],\"packageUris\":[\"http://schema.mathworks.com/mf0/Connector/R2020b\"],\"version\":\"1.0\"}"

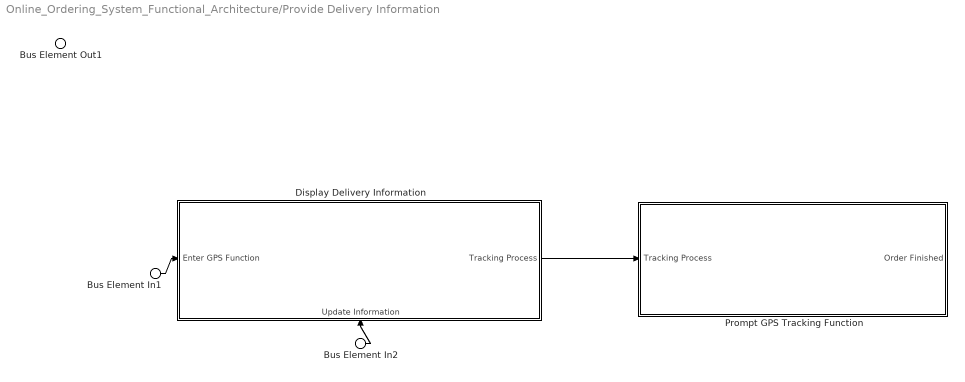
== system Online_Ordering_System_Functional_Architecture/Provide Delivery Information ==
  Bus Element In2 : Inport  PortName=Update Information
  Bus Element In1 : Inport  Port=2  PortName=Enter GPS Function
  Display Delivery Information : Subsystem
      settings: PortSchema="{\"entries\":[{\"content\":{\"headerSize\":26,\"margin\":15,\"minimumSpacing\":25,\"sides\":[{\"content\":{\"connectorIds\":[\"In2\"]},\"type\":\"ConnectorPlacement.EquallySpacedRectSide\",\"uuid\":\"427d1f3e-23ef-431e-830a-8ee80d1c0343\"},{\"content\":{\"connectorIds\":[\"Out1\"],\"side\":\"RIGHT\"},\"type\":\"ConnectorPlacement.EquallySpacedRectSide\",\"uuid\":\"a94733dc-dc80-40b7-a069-e69a5f529ec8\"},{\"content\":{\"side\":\"TOP\"},\"type\":\"ConnectorPlacement.EquallySpacedRectSide\",\"uuid\":\"aab6e856-7d0a-4bba-a547-38d5d593c589\"},{\"content\":{\"connectorIds\":[\"In1\"],\"side\":\"BOTTOM\"},\"type\":\"ConnectorPlacement.EquallySpacedRectSide\",\"uuid\":\"9b163a09-8a4d-4810-a0ad-ac99f601e974\"}]},\"type\":\"ConnectorPlacement.EquallySpacedConnector\",\"uuid\":\"17eb8191-1c5c-46d9-ae9e-c0a8464555a8\"}],\"packageUris\":[\"http://schema.mathworks.com/mf0/Connector/R2020b\"],\"version\":\"1.0\"}"
  Prompt GPS Tracking Function : Subsystem
      settings: PortSchema="{\"entries\":[{\"content\":{\"headerSize\":26,\"margin\":15,\"minimumSpacing\":25,\"sides\":[{\"content\":{\"connectorIds\":[\"In1\"]},\"type\":\"ConnectorPlacement.EquallySpacedRectSide\",\"uuid\":\"427d1f3e-23ef-431e-830a-8ee80d1c0343\"},{\"content\":{\"connectorIds\":[\"Out1\"],\"side\":\"RIGHT\"},\"type\":\"ConnectorPlacement.EquallySpacedRectSide\",\"uuid\":\"a94733dc-dc80-40b7-a069-e69a5f529ec8\"},{\"content\":{\"side\":\"TOP\"},\"type\":\"ConnectorPlacement.EquallySpacedRectSide\",\"uuid\":\"aab6e856-7d0a-4bba-a547-38d5d593c589\"}]},\"type\":\"ConnectorPlacement.EquallySpacedConnector\",\"uuid\":\"17eb8191-1c5c-46d9-ae9e-c0a8464555a8\"}],\"packageUris\":[\"http://schema.mathworks.com/mf0/Connector/R2020b\"],\"version\":\"1.0\"}"
  Bus Element Out1 : Outport  PortName=Order Finished
  wires:
  Display Delivery Information/1(Tracking Process) -> Prompt GPS Tracking Function/1(Tracking Process)
  Bus Element In1/1 -> Display Delivery Information/2(Enter GPS Function)
  Bus Element In2/1 -> Display Delivery Information/1(Update Information)

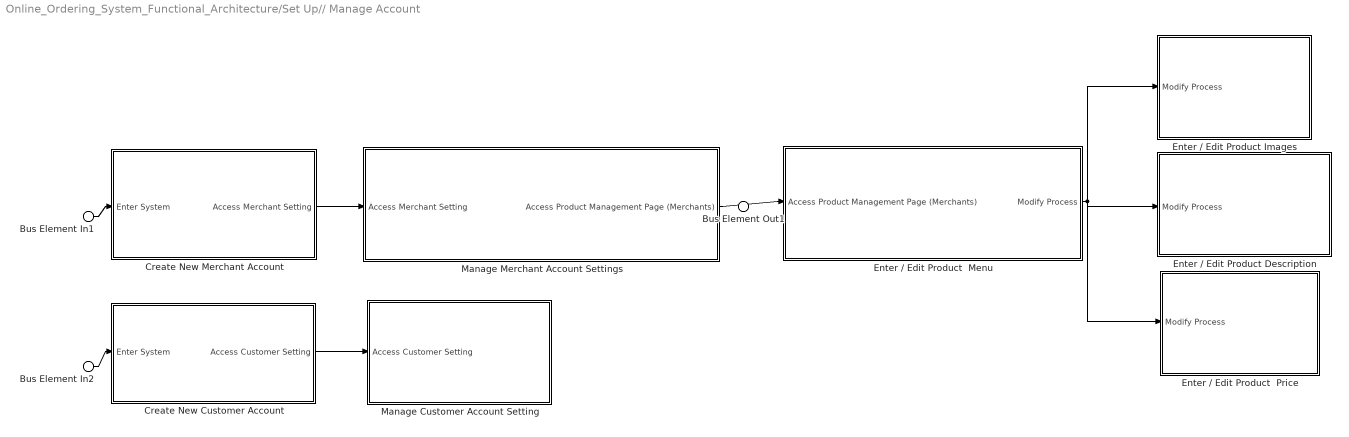
== system Online_Ordering_System_Functional_Architecture/Set Up// Manage Account ==
  Bus Element In1 : Inport  PortName=Enter System
  Bus Element In2 : Inport  PortName=Enter System
  Create New Customer Account : Subsystem
      settings: PortSchema="{\"entries\":[{\"content\":{\"headerSize\":26,\"margin\":15,\"minimumSpacing\":25,\"sides\":[{\"content\":{\"connectorIds\":[\"In1\"]},\"type\":\"ConnectorPlacement.EquallySpacedRectSide\",\"uuid\":\"d2ebed04-42f4-4bd6-aa56-c214d37abe86\"},{\"content\":{\"connectorIds\":[\"Out1\"],\"side\":\"RIGHT\"},\"type\":\"ConnectorPlacement.EquallySpacedRectSide\",\"uuid\":\"0a328130-2da5-4535-b8fd-dee261bd04a3\"},{\"content\":{\"side\":\"TOP\"},\"type\":\"ConnectorPlacement.EquallySpacedRectSide\",\"uuid\":\"410ea5eb-e20b-4523-bb7e-a86253749ceb\"}]},\"type\":\"ConnectorPlacement.EquallySpacedConnector\",\"uuid\":\"5600d62f-d466-4629-981b-50f24b9b11a3\"}],\"packageUris\":[\"http://schema.mathworks.com/mf0/Connector/R2020b\"],\"version\":\"1.0\"}"
  "Create New Merchant Account " : Subsystem
      settings: PortSchema="{\"entries\":[{\"content\":{\"headerSize\":26,\"margin\":15,\"minimumSpacing\":25,\"sides\":[{\"content\":{\"connectorIds\":[\"In1\"]},\"type\":\"ConnectorPlacement.EquallySpacedRectSide\",\"uuid\":\"cbb74984-7595-4789-b046-96ead26edeb9\"},{\"content\":{\"connectorIds\":[\"Out1\"],\"side\":\"RIGHT\"},\"type\":\"ConnectorPlacement.EquallySpacedRectSide\",\"uuid\":\"b6bb8368-8099-4b12-9d55-2c29ae804ffc\"},{\"content\":{\"side\":\"TOP\"},\"type\":\"ConnectorPlacement.EquallySpacedRectSide\",\"uuid\":\"14a6774e-c600-4f70-83e3-a7d0c3cf7479\"}]},\"type\":\"ConnectorPlacement.EquallySpacedConnector\",\"uuid\":\"469ef3cc-c012-4ecc-a677-bf3638dfce1b\"}],\"packageUris\":[\"http://schema.mathworks.com/mf0/Connector/R2020b\"],\"version\":\"1.0\"}"
  Enter / Edit Product  Menu : Subsystem
      settings: PortSchema="{\"entries\":[{\"content\":{\"headerSize\":26,\"margin\":15,\"minimumSpacing\":25,\"sides\":[{\"content\":{\"connectorIds\":[\"In1\"]},\"type\":\"ConnectorPlacement.EquallySpacedRectSide\",\"uuid\":\"47f10906-199a-4fc3-b50f-b8829921055b\"},{\"content\":{\"connectorIds\":[\"Out1\"],\"side\":\"RIGHT\"},\"type\":\"ConnectorPlacement.EquallySpacedRectSide\",\"uuid\":\"92935151-f687-4cd9-918a-4edbdcb1ae87\"},{\"content\":{\"side\":\"TOP\"},\"type\":\"ConnectorPlacement.EquallySpacedRectSide\",\"uuid\":\"015ac99b-8cf7-4451-a810-2c7151c004f5\"}]},\"type\":\"ConnectorPlacement.EquallySpacedConnector\",\"uuid\":\"2d28be76-8335-46d7-935d-5d2731314622\"}],\"packageUris\":[\"http://schema.mathworks.com/mf0/Connector/R2020b\"],\"version\":\"1.0\"}"
  Enter / Edit Product  Price : Subsystem
      settings: PortSchema="{\"entries\":[{\"content\":{\"headerSize\":26,\"margin\":15,\"minimumSpacing\":25,\"sides\":[{\"content\":{\"connectorIds\":[\"In1\"]},\"type\":\"ConnectorPlacement.EquallySpacedRectSide\",\"uuid\":\"47f10906-199a-4fc3-b50f-b8829921055b\"},{\"content\":{\"side\":\"RIGHT\"},\"type\":\"ConnectorPlacement.EquallySpacedRectSide\",\"uuid\":\"92935151-f687-4cd9-918a-4edbdcb1ae87\"},{\"content\":{\"side\":\"TOP\"},\"type\":\"ConnectorPlacement.EquallySpacedRectSide\",\"uuid\":\"015ac99b-8cf7-4451-a810-2c7151c004f5\"}]},\"type\":\"ConnectorPlacement.EquallySpacedConnector\",\"uuid\":\"2d28be76-8335-46d7-935d-5d2731314622\"}],\"packageUris\":[\"http://schema.mathworks.com/mf0/Connector/R2020b\"],\"version\":\"1.0\"}"
  Enter / Edit Product Description : Subsystem
      settings: PortSchema="{\"entries\":[{\"content\":{\"headerSize\":26,\"margin\":15,\"minimumSpacing\":25,\"sides\":[{\"content\":{\"connectorIds\":[\"In1\"]},\"type\":\"ConnectorPlacement.EquallySpacedRectSide\",\"uuid\":\"47f10906-199a-4fc3-b50f-b8829921055b\"},{\"content\":{\"side\":\"RIGHT\"},\"type\":\"ConnectorPlacement.EquallySpacedRectSide\",\"uuid\":\"92935151-f687-4cd9-918a-4edbdcb1ae87\"},{\"content\":{\"side\":\"TOP\"},\"type\":\"ConnectorPlacement.EquallySpacedRectSide\",\"uuid\":\"015ac99b-8cf7-4451-a810-2c7151c004f5\"}]},\"type\":\"ConnectorPlacement.EquallySpacedConnector\",\"uuid\":\"2d28be76-8335-46d7-935d-5d2731314622\"}],\"packageUris\":[\"http://schema.mathworks.com/mf0/Connector/R2020b\"],\"version\":\"1.0\"}"
  Enter / Edit Product Images : Subsystem
      settings: PortSchema="{\"entries\":[{\"content\":{\"headerSize\":26,\"margin\":15,\"minimumSpacing\":25,\"sides\":[{\"content\":{\"connectorIds\":[\"In1\"]},\"type\":\"ConnectorPlacement.EquallySpacedRectSide\",\"uuid\":\"47f10906-199a-4fc3-b50f-b8829921055b\"},{\"content\":{\"side\":\"RIGHT\"},\"type\":\"ConnectorPlacement.EquallySpacedRectSide\",\"uuid\":\"92935151-f687-4cd9-918a-4edbdcb1ae87\"},{\"content\":{\"side\":\"TOP\"},\"type\":\"ConnectorPlacement.EquallySpacedRectSide\",\"uuid\":\"015ac99b-8cf7-4451-a810-2c7151c004f5\"}]},\"type\":\"ConnectorPlacement.EquallySpacedConnector\",\"uuid\":\"2d28be76-8335-46d7-935d-5d2731314622\"}],\"packageUris\":[\"http://schema.mathworks.com/mf0/Connector/R2020b\"],\"version\":\"1.0\"}"
  Manage Customer Account Setting : Subsystem
      settings: PortSchema="{\"entries\":[{\"content\":{\"headerSize\":26,\"margin\":15,\"minimumSpacing\":25,\"sides\":[{\"content\":{\"connectorIds\":[\"In1\"]},\"type\":\"ConnectorPlacement.EquallySpacedRectSide\",\"uuid\":\"d2ebed04-42f4-4bd6-aa56-c214d37abe86\"},{\"content\":{\"side\":\"RIGHT\"},\"type\":\"ConnectorPlacement.EquallySpacedRectSide\",\"uuid\":\"0a328130-2da5-4535-b8fd-dee261bd04a3\"},{\"content\":{\"side\":\"TOP\"},\"type\":\"ConnectorPlacement.EquallySpacedRectSide\",\"uuid\":\"410ea5eb-e20b-4523-bb7e-a86253749ceb\"}]},\"type\":\"ConnectorPlacement.EquallySpacedConnector\",\"uuid\":\"5600d62f-d466-4629-981b-50f24b9b11a3\"}],\"packageUris\":[\"http://schema.mathworks.com/mf0/Connector/R2020b\"],\"version\":\"1.0\"}"
  Manage Merchant Account Settings : Subsystem
      settings: PortSchema="{\"entries\":[{\"content\":{\"headerSize\":26,\"margin\":15,\"minimumSpacing\":25,\"sides\":[{\"content\":{\"connectorIds\":[\"In1\"]},\"type\":\"ConnectorPlacement.EquallySpacedRectSide\",\"uuid\":\"47f10906-199a-4fc3-b50f-b8829921055b\"},{\"content\":{\"connectorIds\":[\"Out1\"],\"side\":\"RIGHT\"},\"type\":\"ConnectorPlacement.EquallySpacedRectSide\",\"uuid\":\"92935151-f687-4cd9-918a-4edbdcb1ae87\"},{\"content\":{\"side\":\"TOP\"},\"type\":\"ConnectorPlacement.EquallySpacedRectSide\",\"uuid\":\"015ac99b-8cf7-4451-a810-2c7151c004f5\"}]},\"type\":\"ConnectorPlacement.EquallySpacedConnector\",\"uuid\":\"2d28be76-8335-46d7-935d-5d2731314622\"}],\"packageUris\":[\"http://schema.mathworks.com/mf0/Connector/R2020b\"],\"version\":\"1.0\"}"
  Bus Element Out1 : Outport  PortName=Authenticate
  wires:
  "Create New Merchant Account "/1(Access Merchant Setting) -> Manage Merchant Account Settings/1(Access Merchant Setting)
  Enter / Edit Product  Menu/1(Modify Process) -> Enter / Edit Product  Price/1(Modify Process), Enter / Edit Product Description/1(Modify Process), Enter / Edit Product Images/1(Modify Process)
  Manage Merchant Account Settings/1(Access Product Management Page (Merchants)) -> Enter / Edit Product  Menu/1(Access Product Management Page (Merchants))
  Create New Customer Account/1(Access Customer Setting) -> Manage Customer Account Setting/1(Access Customer Setting)
  Bus Element In1/1 -> "Create New Merchant Account "/1(Enter System)
  Bus Element In2/1 -> Create New Customer Account/1(Enter System)

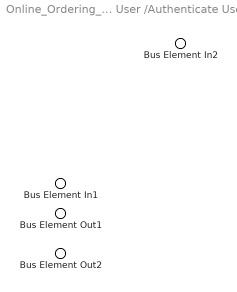
== system Online_Ordering_System_Functional_Architecture/Authenticate User /Authenticate Users ==
  Bus Element In2 : Inport  PortName=Back to Authentication
  Bus Element In1 : Inport  Port=2  PortName=Authenticate Process
  Bus Element Out1 : Outport  PortName=Success
  Bus Element Out2 : Outport  Port=2  PortName=Fail

== system Online_Ordering_System_Functional_Architecture/Authenticate User /Display Login Interface ==
  Bus Element In1 : Inport  PortName=Authenticate
  Bus Element Out1 : Outport  PortName=Enter Account Information

== system Online_Ordering_System_Functional_Architecture/Authenticate User /Prompt a Failed Login ==
  Bus Element In1 : Inport  PortName=Fail
  Bus Element Out1 : Outport  PortName=Back To Login
  Bus Element Out2 : Outport  Port=2  PortName=Back to Authentication

== system Online_Ordering_System_Functional_Architecture/Authenticate User /Sign User In ==
  Bus Element In1 : Inport  PortName=Success
  Bus Element Out2 : Outport  PortName=Enter Homepage

== system Online_Ordering_System_Functional_Architecture/Authenticate User /User Login  ==
  Bus Element In2 : Inport  PortName=Back To Login
  Bus Element In1 : Inport  Port=2  PortName=Enter Account Information
  Bus Element Out1 : Outport  PortName=Authenticate Process

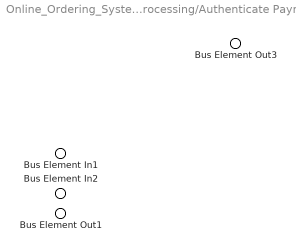
== system Online_Ordering_System_Functional_Architecture/Payment Processing/Authenticate Payment ==
  Bus Element In1 : Inport  PortName=Choose Online Payment
  Bus Element In2 : Inport  Port=2  PortName=Choose Giftcard Payment
  Bus Element Out3 : Outport  PortName=Review Order
  Bus Element Out1 : Outport  Port=2  PortName=Authentication Failure

== system Online_Ordering_System_Functional_Architecture/Payment Processing/Display Payment Confirmation ==
  Bus Element In2 : Inport  PortName=Confirm Order
  Bus Element Out1 : Outport  PortName=Enter GPS Function

== system Online_Ordering_System_Functional_Architecture/Payment Processing/Display Review Order ==
  Bus Element In2 : Inport  PortName=Review Order
  Bus Element Out2 : Outport  PortName=Confirm Order

== system Online_Ordering_System_Functional_Architecture/Payment Processing/Process Gift Card Payment ==
  Bus Element In2 : Inport  PortName=Giftcard
  Bus Element Out1 : Outport  PortName=Choose Giftcard Payment

== system Online_Ordering_System_Functional_Architecture/Payment Processing/Process Online Payment Using CC // DC // Paypal  // Venmo ==
  Bus Element In1 : Inport  PortName=Online
  Bus Element Out1 : Outport  PortName=Choose Online Payment

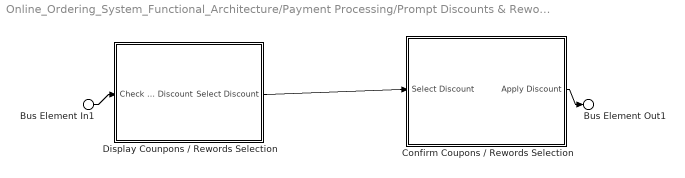
== system Online_Ordering_System_Functional_Architecture/Payment Processing/Prompt Discounts & Rewords ==
  Bus Element In1 : Inport  PortName=Check Out With Discount
  Confirm Coupons / Rewords Selection : Subsystem
      settings: PortSchema="{\"entries\":[{\"content\":{\"headerSize\":26,\"margin\":15,\"minimumSpacing\":25,\"sides\":[{\"content\":{\"connectorIds\":[\"In1\"]},\"type\":\"ConnectorPlacement.EquallySpacedRectSide\",\"uuid\":\"427d1f3e-23ef-431e-830a-8ee80d1c0343\"},{\"content\":{\"connectorIds\":[\"Out1\"],\"side\":\"RIGHT\"},\"type\":\"ConnectorPlacement.EquallySpacedRectSide\",\"uuid\":\"a94733dc-dc80-40b7-a069-e69a5f529ec8\"},{\"content\":{\"side\":\"TOP\"},\"type\":\"ConnectorPlacement.EquallySpacedRectSide\",\"uuid\":\"aab6e856-7d0a-4bba-a547-38d5d593c589\"},{\"content\":{\"side\":\"BOTTOM\"},\"type\":\"ConnectorPlacement.EquallySpacedRectSide\",\"uuid\":\"f7ae7fc0-3d55-4c53-ae74-1880ee28608b\"}]},\"type\":\"ConnectorPlacement.EquallySpacedConnector\",\"uuid\":\"17eb8191-1c5c-46d9-ae9e-c0a8464555a8\"}],\"packageUris\":[\"http://schema.mathworks.com/mf0/Connector/R2020b\"],\"version\":\"1.0\"}"
  Display Counpons / Rewords Selection : Subsystem
      settings: PortSchema="{\"entries\":[{\"content\":{\"headerSize\":26,\"margin\":15,\"minimumSpacing\":25,\"sides\":[{\"content\":{\"connectorIds\":[\"In1\"]},\"type\":\"ConnectorPlacement.EquallySpacedRectSide\",\"uuid\":\"427d1f3e-23ef-431e-830a-8ee80d1c0343\"},{\"content\":{\"connectorIds\":[\"Out1\"],\"side\":\"RIGHT\"},\"type\":\"ConnectorPlacement.EquallySpacedRectSide\",\"uuid\":\"a94733dc-dc80-40b7-a069-e69a5f529ec8\"},{\"content\":{\"side\":\"TOP\"},\"type\":\"ConnectorPlacement.EquallySpacedRectSide\",\"uuid\":\"aab6e856-7d0a-4bba-a547-38d5d593c589\"}]},\"type\":\"ConnectorPlacement.EquallySpacedConnector\",\"uuid\":\"17eb8191-1c5c-46d9-ae9e-c0a8464555a8\"}],\"packageUris\":[\"http://schema.mathworks.com/mf0/Connector/R2020b\"],\"version\":\"1.0\"}"
  Bus Element Out1 : Outport  PortName=Apply Discount
  wires:
  Display Counpons / Rewords Selection/1(Select Discount) -> Confirm Coupons / Rewords Selection/1(Select Discount)
  Bus Element In1/1 -> Display Counpons / Rewords Selection/1(Check Out With Discount)
  Confirm Coupons / Rewords Selection/1(Apply Discount) -> Bus Element Out1/1

== system Online_Ordering_System_Functional_Architecture/Payment Processing/Prompt Payment Methods ==
  Bus Element In2 : Inport  PortName=Check Out Without Discount
  Bus Element In3 : Inport  Port=2  PortName=Apply Discount
  Bus Element In1 : Inport  Port=3  PortName=Authentication Failure
  Bus Element Out1 : Outport  PortName=Selcted Payment Method

== system Online_Ordering_System_Functional_Architecture/Placing Order/Adding To // Remove From Shopping Cart  ==
  Bus Element In5 : Inport  PortName=Go to Shopping Cart
  Bus Element In1 : Inport  Port=2  PortName=Check Shopping Cart
  Bus Element Out1 : Outport  PortName=Finish Add Products

== system Online_Ordering_System_Functional_Architecture/Placing Order/Checking Out From Shopping Cart ==
  Bus Element In1 : Inport  PortName=Finish Add Products
  Bus Element Out1 : Outport  PortName=Check Out

== system Online_Ordering_System_Functional_Architecture/Placing Order/Display Homepage ==
  Bus Element In5 : Inport  PortName=Enter Homepage
  Bus Element Out2 : Outport  PortName=Search / Browsing Product

== system Online_Ordering_System_Functional_Architecture/Placing Order/Display Search Results ==
  Bus Element In2 : Inport  PortName=Select Products by Searching
  Bus Element Out1 : Outport  PortName=Check Shopping Cart

== system Online_Ordering_System_Functional_Architecture/Placing Order/User Products // Stores Browsing Menu ==
  Bus Element In1 : Inport  PortName=Though Browser
  Bus Element Out2 : Outport  PortName=Go to Shopping Cart

== system Online_Ordering_System_Functional_Architecture/Placing Order/User Searching For Product // Stores ==
  Bus Element In1 : Inport  PortName=Though Direct Search
  Bus Element Out1 : Outport  PortName=Select Products by Searching

== system Online_Ordering_System_Functional_Architecture/Process Order /Checking Inventory ==
  Bus Element In1 : Inport  PortName=Checking Availibility
  Bus Element Out1 : Outport  PortName=Pick Up Product From Store
